simulink model "Plant"  (R2025b)
settings: Solver=FixedStepAuto  StartTime=0.0  StopTime=10.0  FixedStep=1e-3  RelTol=1e-3
undefined symbols (not defined in the file or in its folder): cfg
settings Model: Creator=nikol  LastModifiedBy=nikol

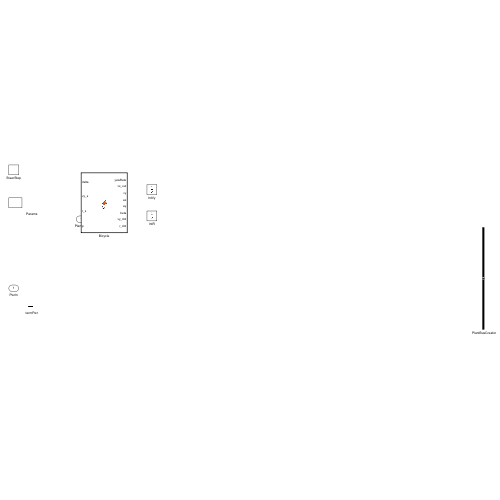
[thumbnail: Simulink's stored preview of the top-level diagram]
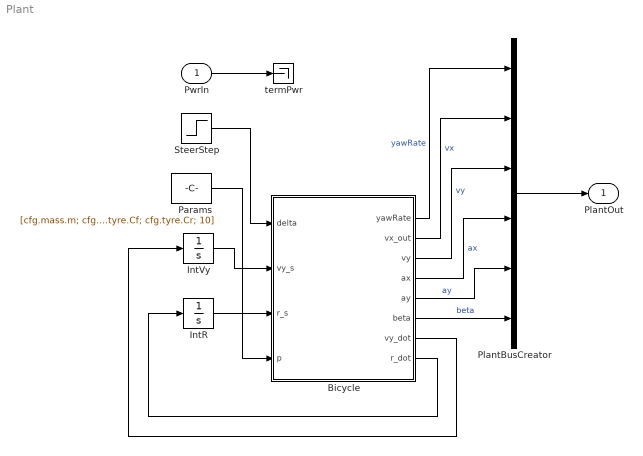
== system Plant ==
  PwrIn : Inport  OutDataTypeStr=Bus: PwrBus
  Bicycle : MATLAB Function  TreatAsAtomicUnit=on
  IntR : Integrator
  IntVy : Integrator
  Params : Constant  Value=[cfg.mass.m; cfg.mass.Iz; cfg.geom.a; cfg.geom.b; cfg.tyre.Cf; cfg.tyre.Cr; 10]
  PlantBusCreator : BusCreator  Inputs=6  OutDataTypeStr=Bus: PlantBus
  SteerStep : Step  After=0.05  SampleTime=0
  termPwr : Terminator
  PlantOut : Outport  OutDataTypeStr=Bus: PlantBus
  wires:
  PwrIn/1 -> termPwr/1
  SteerStep/1 -> Bicycle/1(delta)
  Params/1 -> Bicycle/4(p)
  IntR/1 -> Bicycle/3(r_s)
  IntVy/1 -> Bicycle/2(vy_s)
  Bicycle/1(yawRate) -> PlantBusCreator/1  "yawRate"
  Bicycle/3(vy) -> PlantBusCreator/3  "vy"
  Bicycle/2(vx_out) -> PlantBusCreator/2  "vx"
  Bicycle/4(ax) -> PlantBusCreator/4  "ax"
  Bicycle/5(ay) -> PlantBusCreator/5  "ay"
  Bicycle/6(beta) -> PlantBusCreator/6  "beta"
  Bicycle/7(vy_dot) -> IntVy/1
  Bicycle/8(r_dot) -> IntR/1
  PlantBusCreator/1 -> PlantOut/1

== matlab function Plant/Bicycle ==
  data: delta input; yawRate output; vy_s input; r_s input; p input; vx_out output; vy output; ax output; ay output; beta output; vy_dot output; r_dot output
function [yawRate, vx_out, vy, ax, ay, beta, vy_dot, r_dot] = fcn(delta, vy_s, r_s, p)
    [yawRate, vx_out, vy, ax, ay, beta, vy_dot, r_dot] = bicycleModel(delta, vy_s, r_s, p);
end
